simulink model "DM"  (R2021b)
settings: Solver=VariableStepAuto  StartTime=0.0  StopTime=1  RelTol=1e-3
libraries: commdigbbndpm3 x2, dspfdesign x2, commchan3 x1, commsink2 x1, commrandsrc3 x1
settings Model: Creator=USER  LastModifiedBy=USER

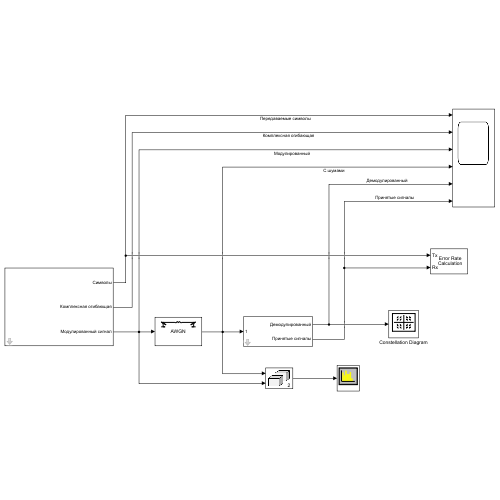
[thumbnail: Simulink's stored preview of the top-level diagram]
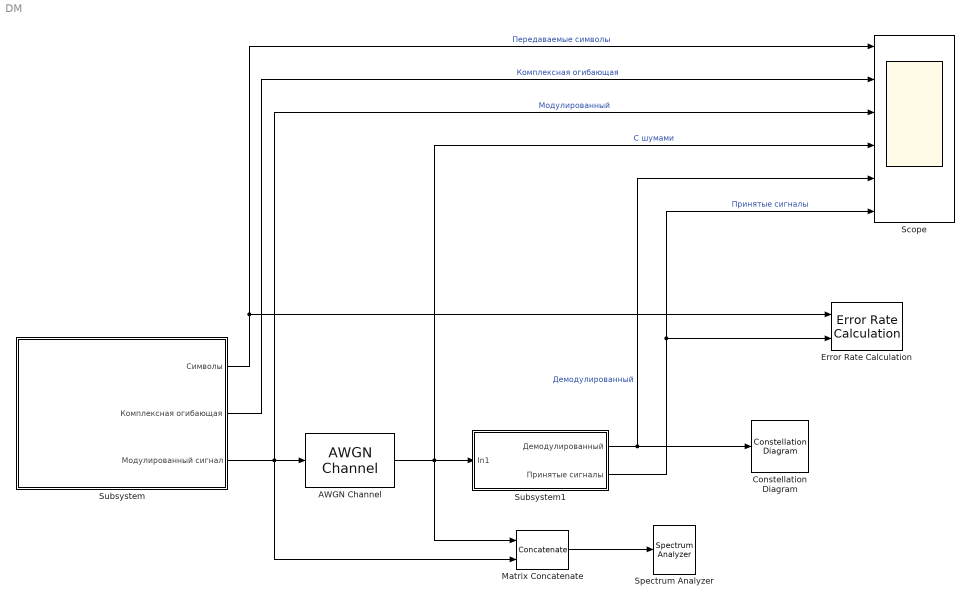
== system DM ==
  AWGN Channel : commchan3/AWGN Channel  InputProcessing=Columns as channels (frame based)  seed=67  noiseMode="Signal to noise ratio  (SNR)"  EbNodB=20  EsNodB=10  SNRdB=20  bitsPerSym=1  Ps=1  Tsym=1  variance=1
  Constellation Diagram : ConstellationDiagram
  Error Rate Calculation : commsink2/Error Rate Calculation  N=1  st_delay=0  cp_mode=Entire frame  subframe=[]  PMode=Workspace  WsName=ErrorVec  RsMode2=off  stop=off  numErr=100  maxBits=1e6
  Matrix Concatenate : Concatenate  Mode=Multidimensional array  ConcatenateDimension=2
  Scope : Scope  NumInputPorts=6
  Spectrum Analyzer : SpectrumAnalyzer
  Subsystem : Subsystem  mask{CarrierFrequency=1e4, SamplingFrequency=1e5, SymbolRate=1e3, size=4}
      mask prompts: CarrierFrequency "Несущая частота"; SamplingFrequency "Частота дискритизации"; SymbolRate "Символьная скорость"; size "Кол-во байт"
  Subsystem1 : Subsystem  mask{CarrierFrequency=1e4, SamplingFrequency=1e5, SymbolRate=1e3, size=4}
      mask prompts: CarrierFrequency "Частота несущей"; SamplingFrequency "Частота дискритизации"; SymbolRate "Символьная скорость"; size "Кол-во байт"
  wires:
  Subsystem/1(Символы) -> Error Rate Calculation/1, Scope/1  "Передаваемые символы"
  Subsystem/2(Комплексная огибающая) -> Scope/2  "Комплексная огибающая"
  Subsystem/3(Модулированный сигнал) -> Matrix Concatenate/2, Scope/3, AWGN Channel/1  "Модулированный"
  AWGN Channel/1 -> Matrix Concatenate/1, Subsystem1/1(In1), Scope/4  "С шумами"
  Subsystem1/1(Демодулированный) -> Constellation Diagram/1, Scope/5  "Демодулированный"
  Subsystem1/2(Принятые сигналы) -> Error Rate Calculation/2, Scope/6  "Принятые сигналы"
  Matrix Concatenate/1 -> Spectrum Analyzer/1

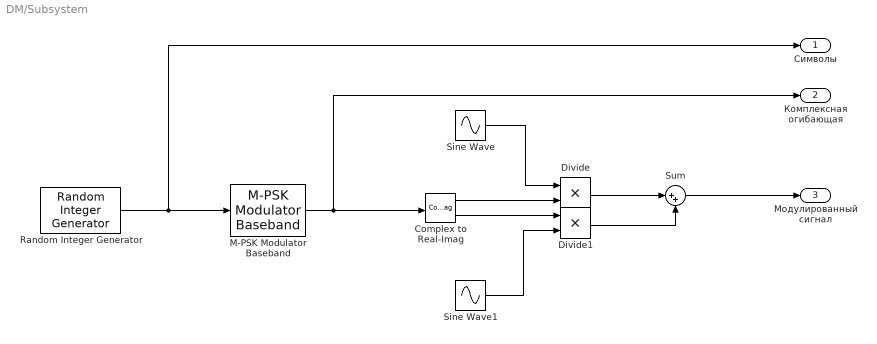
== system DM/Subsystem ==
  Complex to Real-Imag : ComplexToRealImag
  Divide : Product  Inputs=**
  Divide1 : Product  Inputs=**
  M-PSK Modulator Baseband : commdigbbndpm3/M-PSK Modulator Baseband  M=size  InType=Integer  Enc=Gray  Mapping=[0:7]  Ph=pi/8  outDtype=double  outWordLen=16  outUDDataType=sfix(16)  outFracLenMode=Best precision  outFracLen=15  outDataTypeStr=double  outLastDataTypeStr=double
  Random Integer Generator : commrandsrc3/Random Integer Generator  SetSize=size  SeedSource=Auto  Seed=0  SampleTime=1/SymbolRate  SamplesPerFrame=1  OutputDataType=double  SimulateUsing=Interpreted execution
  Sine Wave : Sin  Frequency=2 * pi * CarrierFrequency  SampleTime=1/SamplingFrequency
  Sine Wave1 : Sin  Frequency=1/CarrierFrequency  Phase=pi / 2  SampleTime=1/SamplingFrequency
  Sum : Sum  Inputs=|++
  Символы : Outport
  Комплексная огибающая : Outport  Port=2
  Модулированный сигнал : Outport  Port=3
  wires:
  Random Integer Generator/1 -> Символы/1, M-PSK Modulator Baseband/1
  Sum/1 -> Модулированный сигнал/1
  Sine Wave1/1 -> Divide1/2
  M-PSK Modulator Baseband/1 -> Комплексная огибающая/1, Complex to Real-Imag/1
  Divide/1 -> Sum/1
  Complex to Real-Imag/1 -> Divide/2
  Sine Wave/1 -> Divide/1
  Divide1/1 -> Sum/2
  Complex to Real-Imag/2 -> Divide1/1

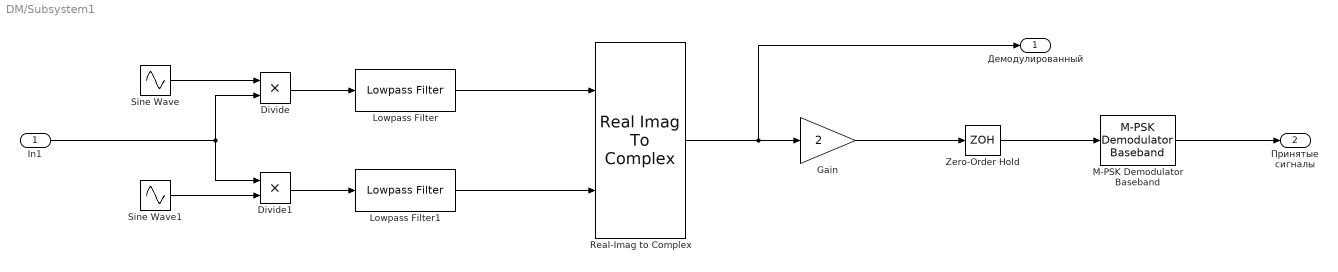
== system DM/Subsystem1 ==
  In1 : Inport
  Divide : Product  Inputs=**
  Divide1 : Product  Inputs=**
  Gain : Gain  Gain=2
  Lowpass Filter : dspfdesign/Lowpass Filter  FilterType=FIR  DesignForMinimumOrder=on  FilterOrder=50  PassbandFrequency=CarrierFrequency  StopbandFrequency=CarrierFrequency * 1.2  PassbandRipple=0.5  StopbandAttenuation=80  InheritSampleRate=on  SampleRate=SamplingFrequency  SimulateUsing=Interpreted execution  roundingMode=Floor  coeffsDataTypeStr=fixdt(1,16)
  Lowpass Filter1 : dspfdesign/Lowpass Filter  FilterType=FIR  DesignForMinimumOrder=on  FilterOrder=50  PassbandFrequency=CarrierFrequency  StopbandFrequency=CarrierFrequency * 1.2  PassbandRipple=0.5  StopbandAttenuation=80  InheritSampleRate=on  SampleRate=SamplingFrequency  SimulateUsing=Interpreted execution  roundingMode=Floor  coeffsDataTypeStr=fixdt(1,16)
  M-PSK Demodulator Baseband : commdigbbndpm3/M-PSK Demodulator Baseband  M=size  OutType=Integer  DecType=Hard decision  VarSource=Dialog  Variance=1  Dec=Gray  Mapping=[0:7]  Ph=pi/4  outDtype1=Inherit via internal rule  outDtype2=Inherit via internal rule  derotateFactorWordLen=16  derotateFactorDataTypeStr=Inherit: Same word length as input  derotateFactorLastDataTypeStr=Inherit: Same word length as input
  Real-Imag to Complex : RealImagToComplex
  Sine Wave : Sin  Frequency=2 * pi * CarrierFrequency  SampleTime=1 / SamplingFrequency
  Sine Wave1 : Sin  Frequency=2 * pi * CarrierFrequency  Phase=pi / 2  SampleTime=1 / SamplingFrequency
  Zero-Order Hold : ZeroOrderHold  SampleTime=1/SymbolRate
  Демодулированный : Outport
  Принятые сигналы : Outport  Port=2
  wires:
  Sine Wave1/1 -> Divide1/2
  Divide1/1 -> Lowpass Filter1/1
  Divide/1 -> Lowpass Filter/1
  Real-Imag to Complex/1 -> Демодулированный/1, Gain/1
  Lowpass Filter/1 -> Real-Imag to Complex/1
  Sine Wave/1 -> Divide/1
  Zero-Order Hold/1 -> M-PSK Demodulator Baseband/1
  M-PSK Demodulator Baseband/1 -> Принятые сигналы/1
  In1/1 -> Divide1/1, Divide/2
  Gain/1 -> Zero-Order Hold/1
  Lowpass Filter1/1 -> Real-Imag to Complex/2
